simulink model "simulim_inverter180"  (R2022b)
settings: Solver=VariableStepAuto  StartTime=0.0  StopTime=10.0  RelTol=1e-3
libraries: spsIGBTLib x6, spsVoltageMeasurementLib x6, spsSeriesRLCBranchLib x3, spsDCVoltageSourceLib x1, sps_lib x1
settings Model: Creator=91894  LastModifiedBy=91894

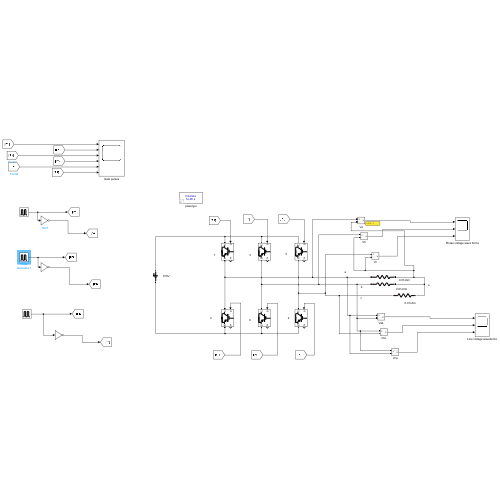
[thumbnail: Simulink's stored preview of the top-level diagram]
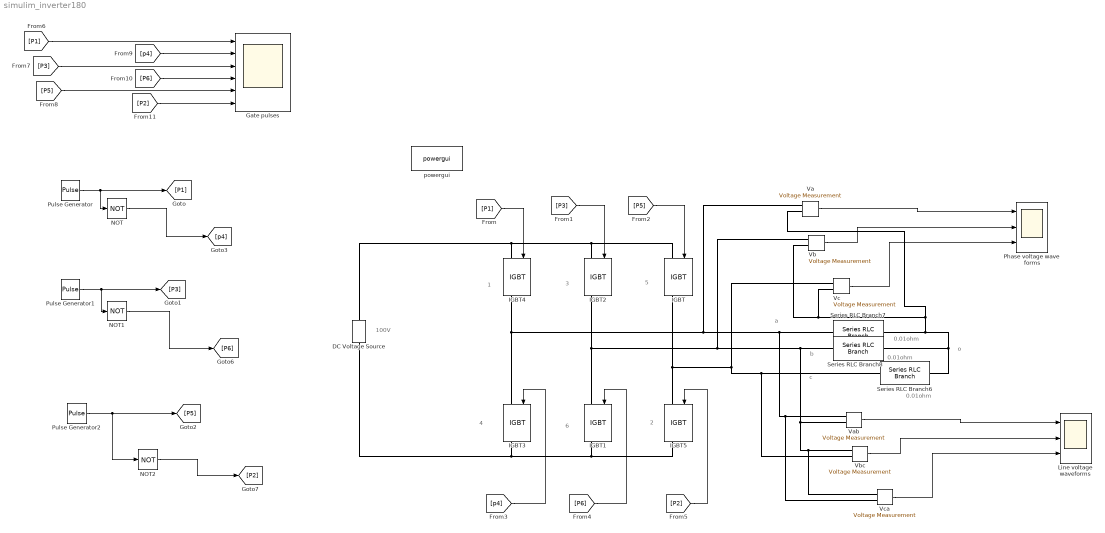
== system simulim_inverter180 ==
  note: 0.01ohm
  note: 100V
  note: c
  note: b
  note: a
  note: o
  note: 2
  note: 1
  note: 3
  note: 4
  note: 6
  note: 5
  note: 0.01ohm
  note: 0.01ohm
  DC Voltage Source : spsDCVoltageSourceLib/DC Voltage Source  Amplitude=100  Measurements=None
  Gate pulses : Scope  NumInputPorts=6
  IGBT{,1..5} (6 alike) : spsIGBTLib/IGBT  Ron=0.001  Lon=0  Vf=1  Tf=1e-6  Tt=2e-6  IC=0  Rs=1e5  Cs=inf  Measurements=on
  Line voltage waveforms : Scope  NumInputPorts=3
  NOT : Logic  Operator=NOT  IconShape=distinctive  AllPortsSameDT=off  OutDataTypeStr=boolean
  NOT1 : Logic  Operator=NOT  IconShape=distinctive  AllPortsSameDT=off  OutDataTypeStr=boolean
  NOT2 : Logic  Operator=NOT  IconShape=distinctive  AllPortsSameDT=off  OutDataTypeStr=boolean
  Phase voltage wave forms : Scope  NumInputPorts=3
  Pulse Generator : DiscretePulseGenerator  PulseType=Time based  Period=1/12000  PulseWidth=50
  Pulse Generator1 : DiscretePulseGenerator  PulseType=Time based  Period=1/12000  PulseWidth=50  PhaseDelay=1/36000
  Pulse Generator2 : DiscretePulseGenerator  PulseType=Time based  Period=1/12000  PulseWidth=50  PhaseDelay=2/36000
  Series RLC Branch6 : spsSeriesRLCBranchLib/Series RLC Branch  LConnTagsString=__new0  RConnTagsString=__new0  BranchType=R  Resistance=0.01  Inductance=1e-3  SetiL0=off  InitialCurrent=0  Capacitance=1e-6  Setx0=off  InitialVoltage=0  Measurements=None
  Series RLC Branch7 : spsSeriesRLCBranchLib/Series RLC Branch  LConnTagsString=__new0  RConnTagsString=__new0  BranchType=R  Resistance=0.01  Inductance=1e-3  SetiL0=off  InitialCurrent=0  Capacitance=1e-6  Setx0=off  InitialVoltage=0  Measurements=None
  Series RLC Branch8 : spsSeriesRLCBranchLib/Series RLC Branch  LConnTagsString=__new0  RConnTagsString=__new0  BranchType=R  Resistance=0.01  Inductance=1e-3  SetiL0=off  InitialCurrent=0  Capacitance=1e-6  Setx0=off  InitialVoltage=0  Measurements=None
  Va : spsVoltageMeasurementLib/Voltage Measurement  PhasorSimulation=off  OutputType=Complex  PSBequivalent=0
  Vab : spsVoltageMeasurementLib/Voltage Measurement  PhasorSimulation=off  OutputType=Complex  PSBequivalent=0
  Vb : spsVoltageMeasurementLib/Voltage Measurement  PhasorSimulation=off  OutputType=Complex  PSBequivalent=0
  Vbc : spsVoltageMeasurementLib/Voltage Measurement  PhasorSimulation=off  OutputType=Complex  PSBequivalent=0
  Vc : spsVoltageMeasurementLib/Voltage Measurement  PhasorSimulation=off  OutputType=Complex  PSBequivalent=0
  Vca : spsVoltageMeasurementLib/Voltage Measurement  PhasorSimulation=off  OutputType=Complex  PSBequivalent=0
  powergui : sps_lib/powergui  Priority=1  SimulationMode=Discrete  SampleTime=1e-6  frequency=60  Iterations=50  frequencyindice=0  Pbase=100e6  ErrMax=1e-4  UnitsV=kV  UnitsW=MW  buscounter=0  FunctionMessages=off  echomessages=off  EnableUseOfTLC=off  CurrentSourceSwitches=off  DisableSnubberDevices=off  DisableRonSwitches=off  DisableVfSwitches=off  DisplayEquations=off  AutomaticDiscreteSolvers=off  SolverType=Tustin/Backward Euler (TBE)  Interpol=off  ExternalGateDelay=off  methode=off  Ts=100  x0status=blocks  SPID=on  SwTol=0  HookPort=off  NonlinearTolerance=1e-4  nMaxIteration=100  ContinueOnMaxIteration=off  RestoreLinks=warning  ResistiveCurrentMeasurement=off  Frange=[0:2:500]  Ylog=off  Xlog=on  ShowGrid=off  save=off  variable=ZData  structure=0  ZoomFFT=off  StartTime=0.0  cycles=1  DisplayStyle=1  fundamental=60  FreqAxis=off  MaxFrequency=1000  frequencyindicesteady=1  RmsSteady=1  display=off
  wires:
  [P6] -> IGBT1/1
  [P5] -> IGBT/1
  Vb/1 -> Phase voltage wave forms/2
  Va/1 -> Phase voltage wave forms/1
  [P1] -> IGBT4/1
  [p4] -> IGBT3/1
  Vc/1 -> Phase voltage wave forms/3
  [P2] -> IGBT5/1
  [P3] -> IGBT2/1
  [P1] -> Gate pulses/1
  [P3] -> Gate pulses/3
  [P5] -> Gate pulses/5
  [p4] -> Gate pulses/2
  [P6] -> Gate pulses/4
  [P2] -> Gate pulses/6
  Pulse Generator/1 -> NOT/1, [P1]
  Pulse Generator1/1 -> NOT1/1, [P3]
  Pulse Generator2/1 -> NOT2/1, [P5]
  NOT/1 -> [p4]
  NOT1/1 -> [P6]
  NOT2/1 -> [P2]
  Vca/1 -> Line voltage waveforms/3
  Vbc/1 -> Line voltage waveforms/2
  Vab/1 -> Line voltage waveforms/1
  connections:
  IGBT1/LConn1 -- IGBT2/RConn1 -- Vca/LConn1 -- Vbc/LConn1 -- Vab/LConn2 -- Series RLC Branch8/LConn1 -- Vb/LConn1
  IGBT5/LConn1 -- IGBT/RConn1 -- Vbc/LConn2 -- Series RLC Branch6/LConn1 -- Vc/LConn1
  DC Voltage Source/RConn1 -- IGBT4/LConn1 -- IGBT2/LConn1 -- IGBT/LConn1
  DC Voltage Source/LConn1 -- IGBT3/RConn1 -- IGBT5/RConn1 -- IGBT1/RConn1
  Va/LConn2 -- Vb/LConn2 -- Vc/LConn2 -- Series RLC Branch8/RConn1 -- Series RLC Branch6/RConn1 -- Series RLC Branch7/RConn1
  IGBT3/LConn1 -- IGBT4/RConn1 -- Vca/LConn2 -- Vab/LConn1 -- Series RLC Branch7/LConn1 -- Va/LConn1
